simulink model "better_model"  (R2022b)
settings: Solver=VariableStepAuto  StartTime=0.0  StopTime=500  RelTol=1e-3
libraries: slpidlib x1
settings Model: Creator=Tyler  LastModifiedBy=Tyler

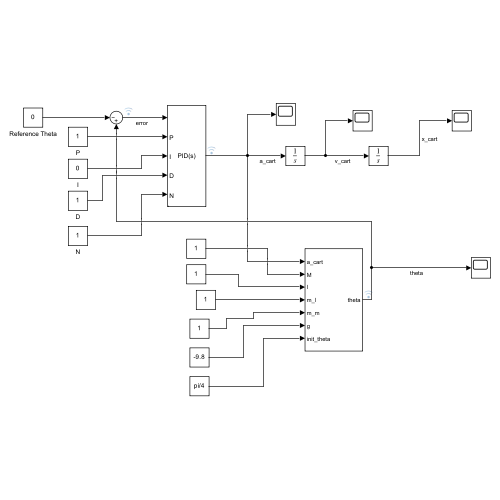
[thumbnail: Simulink's stored preview of the top-level diagram]
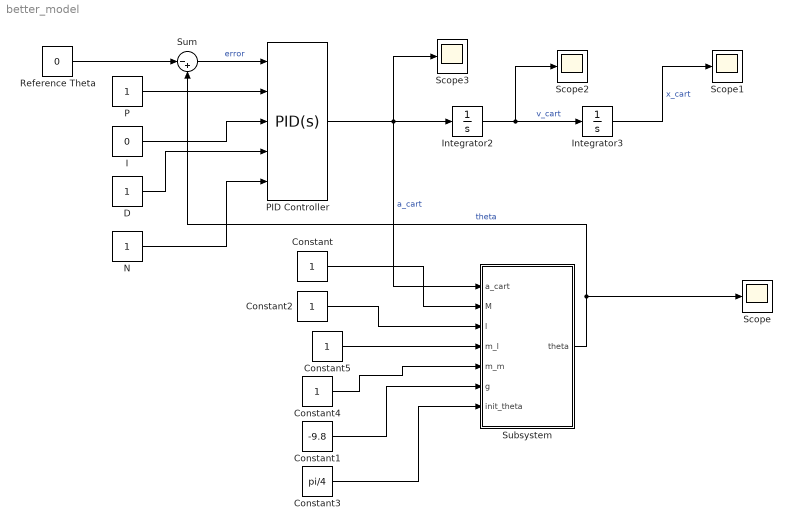
== system better_model ==
  Constant{,2,4..5} (4 alike) : Constant
  Constant1 : Constant  Value=-9.8
  Constant3 : Constant  Value=pi/4
  D : Constant
  I : Constant  Value=0
  Integrator2 : Integrator
  Integrator3 : Integrator  UpperSaturationLimit=3  LowerSaturationLimit=-3
  N : Constant
  P : Constant
  PID Controller : slpidlib/PID Controller  Controller=PID  Form=Parallel  TimeDomain=Continuous-time  UseExternalTs=off  SampleTime=-1  IntegratorMethod=Forward Euler  FilterMethod=Forward Euler  ControllerParametersSource=external  P=0.01  I=0.01  UseKiTs=off  D=0  N=100  UseFilter=on  TunerSelectOption=Transfer Function Based (PID Tuner App)  InitialConditionSource=internal  InitialConditionForIntegrator=0  InitialConditionForFilter=0  DifferentiatorICPrevScaledInput=0  ExternalReset=none  TrackingMode=off  Kt=1  LimitOutput=off  SatLimitsSource=internal  UpperSaturationLimit=1  LowerSaturationLimit=-1  LinearizeAsGain=on  AntiWindupMode=none  Kb=1  LimitIntegrator=off  UpperIntegratorSaturationLimit=inf  LowerIntegratorSaturationLimit=-inf  POutMin=[]  POutMax=[]  IOutMin=[]  IOutMax=[]  DOutMin=[]  DOutMax=[]  NOutMin=[]  NOutMax=[]  SumOutMin=[]  SumOutMax=[]  SaturationOutMin=[]  SaturationOutMax=[]  PParamMin=[]  PParamMax=[]  IParamMin=[]  IParamMax=[]  DParamMin=[]  DParamMax=[]  NParamMin=[]  NParamMax=[]  KbParamMin=[]  KbParamMax=[]  KtParamMin=[]  KtParamMax=[]  KbOutMin=[]  KbOutMax=[]  KtOutMin=[]  KtOutMax=[]  IntegratorOutMin=[]  IntegratorOutMax=[]  FilterOutMin=[]  FilterOutMax=[]  SumI1OutMin=[]  SumI1OutMax=[]  SumI2OutMin=[]  SumI2OutMax=[]  SumI3OutMin=[]  SumI3OutMax=[]  SumI4OutMin=[]  SumI4OutMax=[]  SumDOutMin=[]  SumDOutMax=[]  DifferentiatorOutMin=[]  DifferentiatorOutMax=[]  FilterDiffOutCoefMin=[]  FilterDiffOutCoefMax=[]  ReciprocalOutMin=[]  ReciprocalOutMax=[]  SumDenOutMin=[]  SumDenOutMax=[]  SumNumOutMin=[]  SumNumOutMax=[]  DivideOutMin=[]  DivideOutMax=[]  UdiffTsProdOutMin=[]  UdiffTsProdOutMax=[]  NTsProdOutMin=[]  NTsProdOutMax=[]  UintegralTsProdOutMin=[]  UintegralTsProdOutMax=[]  UngainTsProdOutMin=[]  UngainTsProdOutMax=[]  ClampingZeroOutDataTypeStr=Inherit: Inherit via back propagation  ClampingZeroOutMin=[]  ClampingZeroOutMax=[]  FilterDenConstantOutDataTypeStr=Inherit: Inherit via back propagation  FilterDenConstantOutMin=[]  FilterDenConstantOutMax=[]  PCopyOutDataTypeStr=Inherit: Inherit via back propagation  PCopyOutMin=[]  PCopyOutMax=[]  NCopyOutDataTypeStr=Inherit: Inherit via back propagation  NCopyOutMin=[]  NCopyOutMax=[]  IntegratorContinuousStateAttributes=''  IntegratorStateMustResolveToSignalObject=off  IntegratorRTWStateStorageClass=Auto  FilterContinuousStateAttributes=''  FilterStateMustResolveToSignalObject=off  FilterRTWStateStorageClass=Auto  ParallelPVariant=ExternalParameters  IdealPVariant=Disabled  IVariant=ExternalParameters  DVariant=ExternalParameters  IntegratorVariant=Continuous  SatVariant=Disabled  AWVariant=Passthrough  PCopyVariant=Disabled  TRVariant=Disabled  FdbkBlocksVariant=Forward  IdealPFdbkVariant=Disabled  SatFdbkVariant=Disabled  DerivativeFilterVariant=ContFilter  NVariant=ExternalParameters  NCopyVariant=Disabled  FilterICVariant=InternalICsFilter  IntegratorICVariant=InternalICs  ExternalResetVariant=Disabled  TRSumVariant=Passthrough  SumFdbkVariant=Disabled  SumVariant=Sum_PID  TsampFilterVariant=InternalTs  TsampNgainVariant=Passthrough  TsampIntegralVariant=Passthrough  ExternalSaturationOutDataTypeStr=Inherit: Same as second input
  Reference Theta : Constant  Value=0
  Scope{,1..3} (4 alike) : Scope
  Subsystem : Subsystem
  Sum : Sum  Inputs=|-+
  wires:
  N/1 -> PID Controller/5
  Reference Theta/1 -> Sum/1
  Subsystem/1(theta) -> Scope/1, Sum/2  "theta"
  Constant4/1 -> Subsystem/5(m_m)
  Constant3/1 -> Subsystem/7(init_theta)
  I/1 -> PID Controller/3
  Constant2/1 -> Subsystem/3(l)
  Integrator3/1 -> Scope1/1  "x_cart"
  Constant/1 -> Subsystem/2(M)
  Constant1/1 -> Subsystem/6(g)
  Sum/1 -> PID Controller/1  "error"
  P/1 -> PID Controller/2
  Integrator2/1 -> Integrator3/1, Scope2/1  "v_cart"
  D/1 -> PID Controller/4
  PID Controller/1 -> Subsystem/1(a_cart), Integrator2/1, Scope3/1  "a_cart"
  Constant5/1 -> Subsystem/4(m_l)

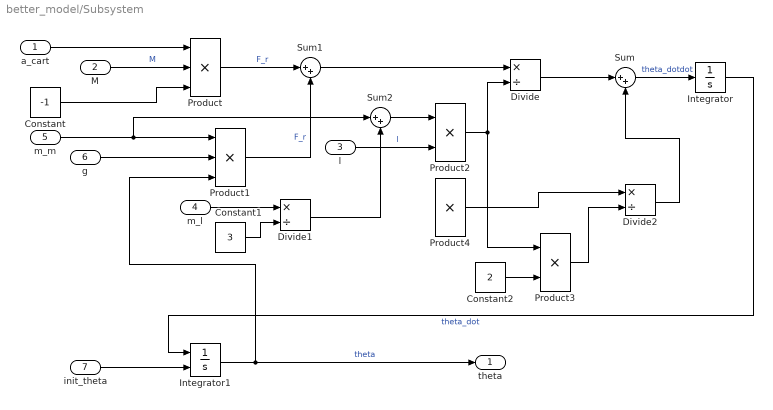
== system better_model/Subsystem ==
  a_cart : Inport
  M : Inport  Port=2
  l : Inport  Port=3
  m_l : Inport  Port=4
  m_m : Inport  Port=5
  g : Inport  Port=6
  init_theta : Inport  Port=7
  Constant : Constant  Value=-1
  Constant1 : Constant  Value=3
  Constant2 : Constant  Value=2
  Divide : Product  Inputs=*/
  Divide1 : Product  Inputs=*/
  Divide2 : Product  Inputs=*/
  Integrator : Integrator
  Integrator1 : Integrator  InitialConditionSource=external  InitialCondition=pi  LimitOutput=on  UpperSaturationLimit=pi  LowerSaturationLimit=-pi
  Product : Product  Inputs=3
  Product1 : Product  Inputs=3
  Product2 : Product
  Product3 : Product
  Product4 : Product  Inputs=3
  Sum : Sum  Inputs=|++
  Sum1 : Sum  Inputs=|++
  Sum2 : Sum  Inputs=|++
  theta : Outport
  wires:
  Sum/1 -> Integrator/1  "theta_dotdot"
  Integrator1/1 -> theta/1, Product1/3  "theta"
  a_cart/1 -> Product/1
  Integrator/1 -> Integrator1/1  "theta_dot"
  M/1 -> Product/2  "M"
  init_theta/1 -> Integrator1/2
  Constant/1 -> Product/3
  Product/1 -> Sum1/1  "F_r"
  m_m/1 -> Sum2/1, Product1/1
  g/1 -> Product1/2
  Product1/1 -> Sum1/2  "F_r"
  Sum1/1 -> Divide/1
  m_l/1 -> Divide1/1
  Constant1/1 -> Divide1/2
  Divide/1 -> Sum/1
  l/1 -> Product2/2  "l"
  Constant2/1 -> Product3/2
  Divide2/1 -> Sum/2
  Product3/1 -> Divide2/2
  Divide1/1 -> Sum2/2
  Sum2/1 -> Product2/1
  Product2/1 -> Divide/2, Product3/1
  Product4/1 -> Divide2/1
